simulink model "unitTestCalcMinDist"  (R2018b)
settings: Solver=VariableStepAuto  StartTime=0.0  StopTime=10.0  RelTol=1e-3
libraries: BasicAircraftDynamicsBlock x2, CalcMinDist x2, NominalTrajectory x2
settings Model: Creator=PE29732  LastModifiedBy=BI28030

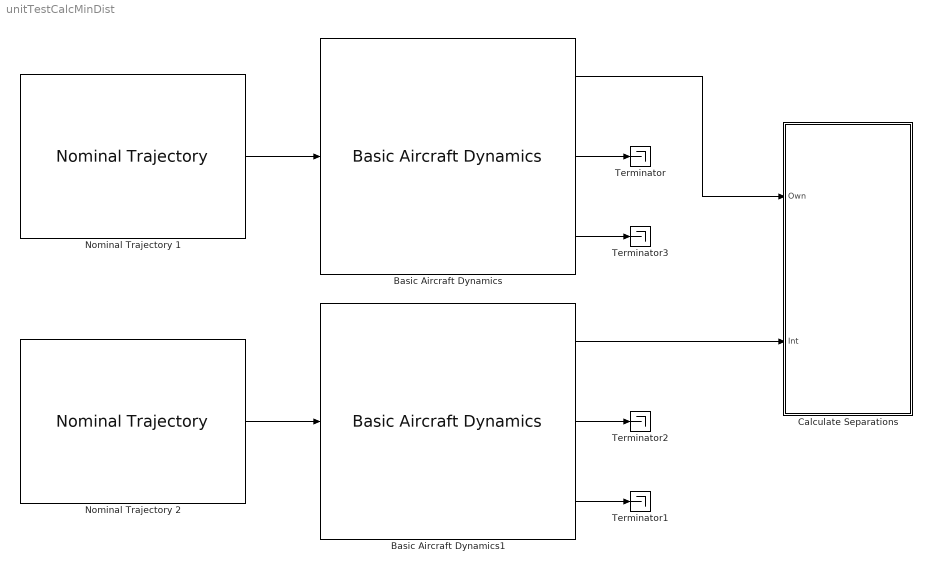
== system unitTestCalcMinDist ==
  Basic Aircraft Dynamics : BasicAircraftDynamicsBlock/Basic Aircraft Dynamics  ts_dynamics=.1  v_ftps_0=ac1dyn_v_ftps  N_ft_0=ac1dyn_N_ft  E_ft_0=ac1dyn_E_ft  h_ft_0=ac1dyn_h_ft  psi_rad_0=ac1dyn_psi_rad  theta_rad_0=ac1dyn_theta_rad  phi_rad_0=ac1dyn_phi_rad  a_ftpss_0=ac1dyn_a_ftpss  v_ftps_max=ac1dyn_con.maxAirspeed_ftps  v_ftps_min=ac1dyn_con.minAirspeed_ftps  dv_ftpss_max=ac1dyn_con.maxAcceleration_ftpss  dv_ftpss_min=ac1dyn_con.minAcceleration_ftpss  dh_ftps_max=ac1dyn_con.maxVerticalRate_ftps  dh_ftps_min=ac1dyn_con.minVerticalRate_ftps  q_radps_max=ac1dyn_con.maxPitchRate_radps  phi_rad_max=ac1dyn_con.maxBankAngle_rad  dphi_radps_max=ac1dyn_con.maxRollRate_radps  r_radps_max=ac1dyn_con.maxYawRate_radps  pNUM=ac1dyn_con.dynamicsNumeratorRollRate  pDEN=ac1dyn_con.dynamicsDenominatorRollRate  hNUM=ac1dyn_con.dynamicsNumeratorVerticalRate  hDEN=ac1dyn_con.dynamicsDenominatorVerticalRate  rNUM=ac1dyn_con.dynamicsNumeratorYawRate  rDEN=ac1dyn_con.dynamicsDenominatorYawRate  lat0_rad=ac2dyn_lat0_rad  lon0_rad=ac2dyn_lon0_rad  alt_ft=ac2dyn_alt0_ft
  Basic Aircraft Dynamics1 : BasicAircraftDynamicsBlock/Basic Aircraft Dynamics  ts_dynamics=.1  v_ftps_0=ac2dyn_v_ftps  N_ft_0=ac2dyn_N_ft  E_ft_0=ac2dyn_E_ft  h_ft_0=ac2dyn_h_ft  psi_rad_0=ac2dyn_psi_rad  theta_rad_0=ac2dyn_theta_rad  phi_rad_0=ac2dyn_phi_rad  a_ftpss_0=ac2dyn_a_ftpss  v_ftps_max=ac2dyn_con.maxAirspeed_ftps  v_ftps_min=ac2dyn_con.minAirspeed_ftps  dv_ftpss_max=ac2dyn_con.maxAcceleration_ftpss  dv_ftpss_min=ac2dyn_con.minAcceleration_ftpss  dh_ftps_max=ac2dyn_con.maxVerticalRate_ftps  dh_ftps_min=ac2dyn_con.minVerticalRate_ftps  q_radps_max=ac2dyn_con.maxPitchRate_radps  phi_rad_max=ac2dyn_con.maxBankAngle_rad  dphi_radps_max=ac2dyn_con.maxRollRate_radps  r_radps_max=ac2dyn_con.maxYawRate_radps  pNUM=ac2dyn_con.dynamicsNumeratorRollRate  pDEN=ac2dyn_con.dynamicsDenominatorRollRate  hNUM=ac2dyn_con.dynamicsNumeratorVerticalRate  hDEN=ac2dyn_con.dynamicsDenominatorVerticalRate  rNUM=ac2dyn_con.dynamicsNumeratorYawRate  rDEN=ac2dyn_con.dynamicsDenominatorYawRate  lat0_rad=ac2dyn_lat0_rad  lon0_rad=ac2dyn_lon0_rad  alt_ft=ac2dyn_alt0_ft
  Calculate Separations : Subsystem  AncestorBlock=CommonMetrics/Common Metrics/Calculate Separations
  Nominal Trajectory 1 : NominalTrajectory/Nominal Trajectory  eventFilename=event1.mat  ts=.1
  Nominal Trajectory 2 : NominalTrajectory/Nominal Trajectory  eventFilename=event2.mat  ts=.1
  Terminator{,1..3} (4 alike) : Terminator
  wires:
  Nominal Trajectory 2/1 -> Basic Aircraft Dynamics1/1
  Basic Aircraft Dynamics/3 -> Terminator3/1
  Nominal Trajectory 1/1 -> Basic Aircraft Dynamics/1
  Basic Aircraft Dynamics1/3 -> Terminator1/1
  Basic Aircraft Dynamics/2 -> Terminator/1
  Basic Aircraft Dynamics1/2 -> Terminator2/1
  Basic Aircraft Dynamics/1 -> Calculate Separations/1(Own)
  Basic Aircraft Dynamics1/1 -> Calculate Separations/2(Int)

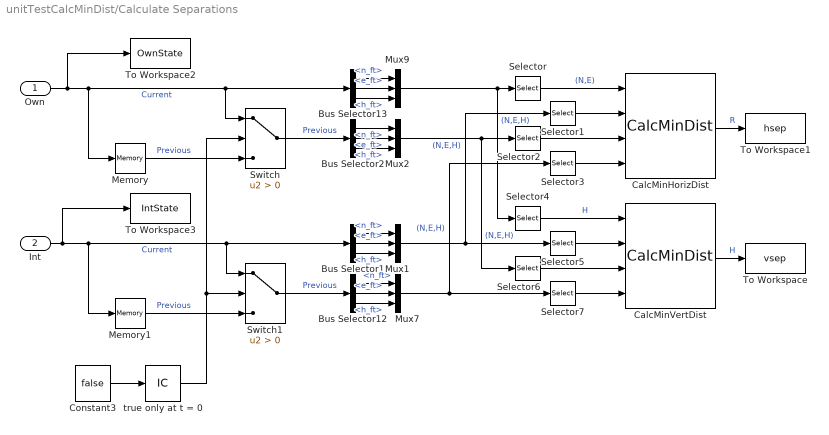
== system unitTestCalcMinDist/Calculate Separations ==
  Own : Inport
  Int : Inport  Port=2
  Bus Selector{1..2,12..13} (4 alike) : BusSelector  OutputSignals=n_ft,e_ft,h_ft
  CalcMinHorizDist : CalcMinDist/CalcMinDist
      settings: SourceProductName=CASSATTv6: Metrics Library
  CalcMinVertDist : CalcMinDist/CalcMinDist
      settings: SourceProductName=CASSATTv6: Metrics Library
  Constant3 : Constant  Value=false  SampleTime=Inf
  Memory : Memory
  Memory1 : Memory
  Mux{1..2,7,9} (4 alike) : Mux  Inputs=3
  Selector{,1..3} (4 alike) : Selector  InputPortWidth=3  IndexOptions=Index vector (dialog)  Indices=[1 2]  OutputSizes=1
  Selector{4..7} (4 alike) : Selector  InputPortWidth=3  IndexOptions=Index vector (dialog)  Indices=3  OutputSizes=1
  Switch : Switch  Criteria=u2 > Threshold
  Switch1 : Switch  Criteria=u2 > Threshold
  To Workspace : ToWorkspace  VariableName=vsep  SaveFormat=Timeseries  SampleTime=-1
  To Workspace1 : ToWorkspace  VariableName=hsep  SaveFormat=Timeseries  SampleTime=-1
  To Workspace2 : ToWorkspace  VariableName=OwnState  SaveFormat=Timeseries  SampleTime=-1
  To Workspace3 : ToWorkspace  VariableName=IntState  SaveFormat=Timeseries  SampleTime=-1
  true only at t = 0 : InitialCondition  Value=true
  wires:
  CalcMinHorizDist/1 -> To Workspace1/1  "R"
  true only at t = 0/1 -> Switch/2, Switch1/2
  Constant3/1 -> true only at t = 0/1
  Memory1/1 -> Switch1/3  "Previous"
  Memory/1 -> Switch/3  "Previous"
  Mux9/1 -> Selector/1, Selector4/1  "(N,E,H)"
  Bus Selector12/2 -> Mux7/2  "<e_ft>"
  Bus Selector12/1 -> Mux7/1  "<n_ft>"
  Bus Selector12/3 -> Mux7/3  "<h_ft>"
  Mux7/1 -> Selector3/1, Selector7/1  "(N,E,H)"
  Own/1 -> To Workspace2/1, Memory/1, Bus Selector13/1, Switch/1  "Current"
  Switch1/1 -> Bus Selector12/1  "Previous"
  CalcMinVertDist/1 -> To Workspace/1  "H"
  Bus Selector13/1 -> Mux9/1  "<n_ft>"
  Bus Selector13/2 -> Mux9/2  "<e_ft>"
  Bus Selector13/3 -> Mux9/3  "<h_ft>"
  Bus Selector1/1 -> Mux1/1  "<n_ft>"
  Bus Selector1/2 -> Mux1/2  "<e_ft>"
  Bus Selector1/3 -> Mux1/3  "<h_ft>"
  Switch/1 -> Bus Selector2/1  "Previous"
  Bus Selector2/1 -> Mux2/1  "<n_ft>"
  Bus Selector2/2 -> Mux2/2  "<e_ft>"
  Bus Selector2/3 -> Mux2/3  "<h_ft>"
  Mux1/1 -> Selector1/1, Selector5/1  "(N,E,H)"
  Mux2/1 -> Selector6/1, Selector2/1  "(N,E,H)"
  Selector/1 -> CalcMinHorizDist/1  "(N,E)"
  Selector1/1 -> CalcMinHorizDist/2
  Selector2/1 -> CalcMinHorizDist/3
  Selector3/1 -> CalcMinHorizDist/4
  Selector4/1 -> CalcMinVertDist/1  "H"
  Selector5/1 -> CalcMinVertDist/2
  Selector6/1 -> CalcMinVertDist/3
  Selector7/1 -> CalcMinVertDist/4
  Int/1 -> To Workspace3/1, Bus Selector1/1, Switch1/1, Memory1/1  "Current"
